simulink subsystem "HighLevelController"  (R2023a)
settings: Solver=VariableStepAuto  StartTime=0.0  StopTime=10.0  RelTol=1e-3
model mask{PID_P=1, PID_I=1, PID_D=1}
  mask prompts: PID_P "Proportional coeff"; PID_I "Integral coeff"; PID_D "Differential coeff"
settings Model: Creator=user  LastModifiedBy=user

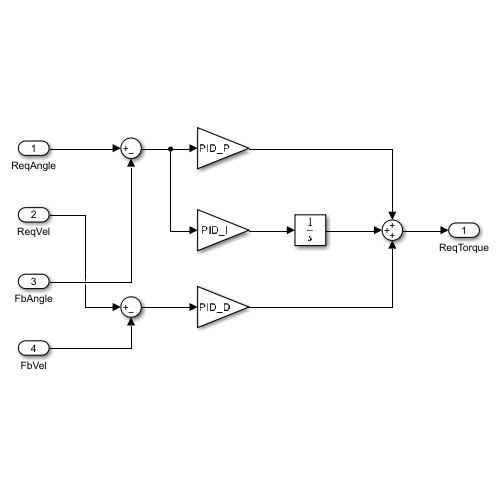
[thumbnail: Simulink's stored preview of the top-level diagram]
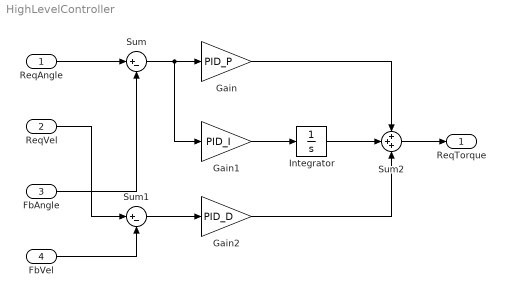
== system HighLevelController ==
  ReqAngle : Inport
  ReqVel : Inport  Port=2
  FbAngle : Inport  Port=3
  FbVel : Inport  Port=4
  Gain : Gain  Gain=PID_P
  Gain1 : Gain  Gain=PID_I
  Gain2 : Gain  Gain=PID_D
  Integrator : Integrator
  Sum : Sum  Inputs=|+-
  Sum1 : Sum  Inputs=|+-
  Sum2 : Sum  Inputs=+++
  ReqTorque : Outport
  wires:
  ReqAngle/1 -> Sum/1
  Sum/1 -> Gain1/1, Gain/1
  Sum2/1 -> ReqTorque/1
  FbAngle/1 -> Sum/2
  ReqVel/1 -> Sum1/1
  FbVel/1 -> Sum1/2
  Gain1/1 -> Integrator/1
  Sum1/1 -> Gain2/1
  Gain2/1 -> Sum2/3
  Integrator/1 -> Sum2/2
  Gain/1 -> Sum2/1
